simulink model "Linearization"  (R2023b)
settings: Solver=VariableStepAuto  StartTime=0.0  StopTime=10.0  RelTol=1e-3
values from neighbouring files (symbols this model uses):
  K1 = 30    [matlab.mat]
  K2 = 20000    [matlab.mat]
  Kd = 2.8    [matlab.mat]
  Kf = 0.00063    [matlab.mat]
  m1 = 0.7    [matlab.mat]
  m2 = 0.3    [matlab.mat]
undefined symbols (not defined in the file or in its folder): linsys1
libraries: cstblocks x4
settings Model: Creator=au756794  LastModifiedBy=JesperBertelsen

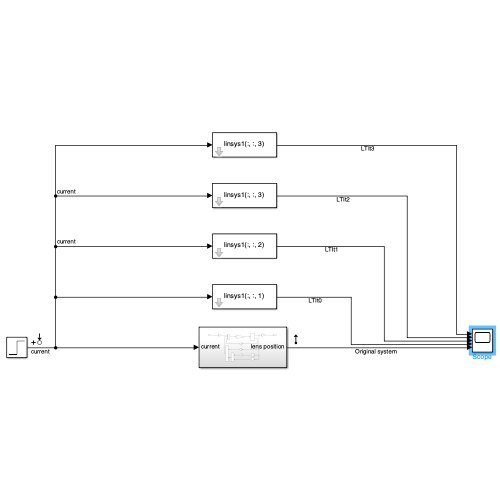
[thumbnail: Simulink's stored preview of the top-level diagram]
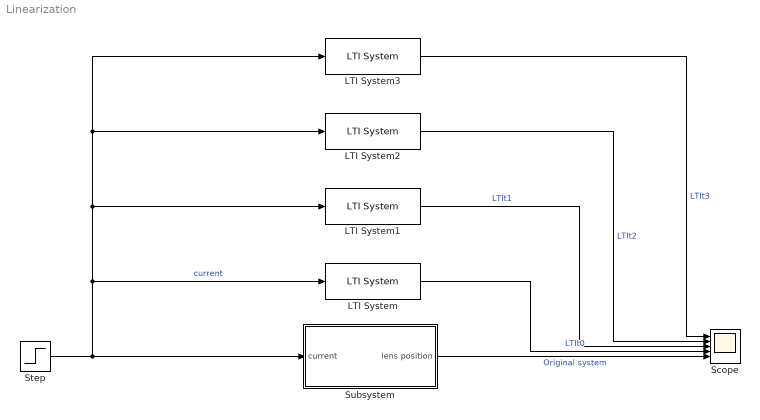
== system Linearization ==
  LTI System : cstblocks/LTI System  sys=linsys1(:, :, 1)  IC=[]  PadeOrder=0
  LTI System1 : cstblocks/LTI System  sys=linsys1(:, :, 2)  IC=[]  PadeOrder=0
  LTI System2 : cstblocks/LTI System  sys=linsys1(:, :, 3)  IC=[]  PadeOrder=0
  LTI System3 : cstblocks/LTI System  sys=linsys1(:, :, 3)  IC=[]  PadeOrder=0
  Scope : Scope  NumInputPorts=5
  Step : Step  SampleTime=0
  Subsystem : Subsystem
  wires:
  Subsystem/1(lens position) -> Scope/5  "Original system"
  Step/1 -> LTI System3/1, LTI System2/1, LTI System1/1, LTI System/1, Subsystem/1(current)  "current"
  LTI System/1 -> Scope/4  "LTIt0"
  LTI System1/1 -> Scope/3  "LTIt1"
  LTI System2/1 -> Scope/2  "LTIt2"
  LTI System3/1 -> Scope/1  "LTIt3"

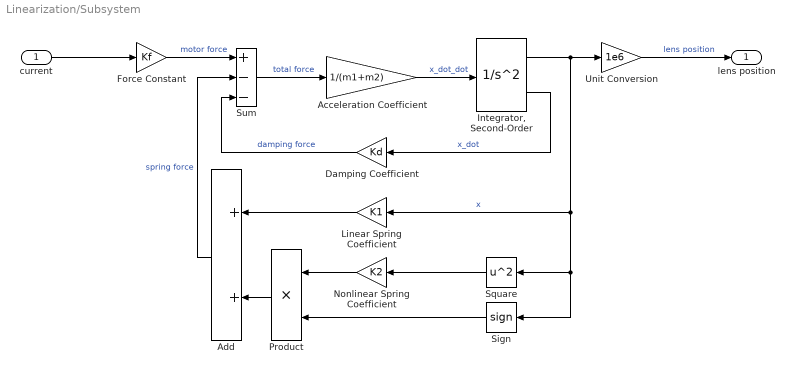
== system Linearization/Subsystem ==
  current : Inport
  Acceleration Coefficient : Gain  Gain=1/(m1+m2)
  Add : Sum
  Damping Coefficient : Gain  Gain=Kd
  Force Constant : Gain  Gain=Kf
  "Integrator, Second-Order" : SecondOrderIntegrator  ICX=0  LimitX=on  UpperLimitX=1e-3  LowerLimitX=0  IgnoreStateLimitsAndResetForLinearization=on
  Linear Spring Coefficient : Gain  Gain=K1
  Nonlinear Spring Coefficient : Gain  Gain=K2
  Product : Product
  Sign : Signum
  Square : Math  Operator=square
  Sum : Sum  Inputs=+--
  Unit Conversion : Gain  Gain=1e6
  lens position : Outport
  wires:
  Unit Conversion/1 -> lens position/1  "lens position"
  Damping Coefficient/1 -> Sum/3  "damping force"
  Nonlinear Spring Coefficient/1 -> Product/1
  Add/1 -> Sum/2  "spring force"
  Force Constant/1 -> Sum/1  "motor force"
  Linear Spring Coefficient/1 -> Add/1
  "Integrator, Second-Order"/2 -> Damping Coefficient/1  "x_dot"
  Product/1 -> Add/2
  Square/1 -> Nonlinear Spring Coefficient/1
  current/1 -> Force Constant/1
  "Integrator, Second-Order"/1 -> Linear Spring Coefficient/1, Square/1, Sign/1, Unit Conversion/1  "x"
  Sum/1 -> Acceleration Coefficient/1  "total force"
  Acceleration Coefficient/1 -> "Integrator, Second-Order"/1  "x_dot_dot"
  Sign/1 -> Product/2
